simulink model "four"  (R2019b)
settings: Solver=VariableStepAuto  StartTime=0.0  StopTime=2  RelTol=1e-3
undefined symbols (not defined in the file): magnitude
libraries: dsparch4 x1
settings Model: Creator=Lenovo  LastModifiedBy=Lenovo

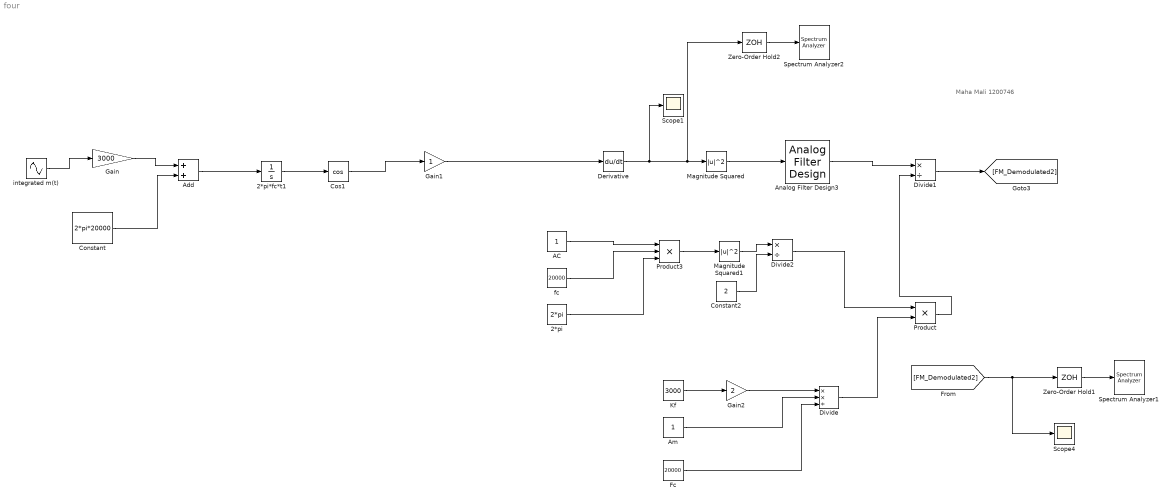
== system four ==
  note: Maha Mali 1200746
  2*pi : Constant  Value=2*pi
  2*pi*fc*t1 : Integrator
  AC : Constant
  Add : Sum
  Am : Constant
  Analog Filter Design3 : dsparch4/Analog Filter Design  method=Butterworth  filttype=Bandpass  N=8  Wlo=pi*2*400  Whi=pi*2*600  Rp=2  Rs=40
  Constant : Constant  Value=2*pi*20000
  Constant2 : Constant  Value=2
  Cos1 : Trigonometry  Operator=cos
  Derivative : Derivative
  Divide : Product  Inputs=**/
  Divide1 : Product  Inputs=*/
  Divide2 : Product  Inputs=*/
  Fc : Constant  Value=20000
  Gain : Gain  Gain=3000
  Gain1 : Gain
  Gain2 : Gain  Gain=2
  Kf : Constant  Value=3000
  Magnitude Squared : Math  Operator=magnitude^2  SignedPower=off  SaturateOnIntegerOverflow=on
  Magnitude Squared1 : Math  Operator=magnitude^2  SignedPower=off  SaturateOnIntegerOverflow=on
  Product : Product
  Product3 : Product  Inputs=3
  Scope1 : Scope
  Scope4 : Scope
  Spectrum Analyzer1 : SpectrumAnalyzer
  Spectrum Analyzer2 : SpectrumAnalyzer
  Zero-Order Hold1 : ZeroOrderHold  SampleTime=1/(10*5e2)
  Zero-Order Hold2 : ZeroOrderHold  SampleTime=1/(10*2e4)
  fc : Constant  Value=20000
  integrated m(t) : Sin  Frequency=500*pi*2  SampleTime=0
  wires:
  Product/1 -> Divide1/2
  Divide1/1 -> [FM_Demodulated2]
  fc/1 -> Product3/2
  Divide2/1 -> Product/1
  Fc/1 -> Divide/3
  Am/1 -> Divide/2
  [FM_Demodulated2] -> Zero-Order Hold1/1, Scope4/1
  AC/1 -> Product3/1
  Kf/1 -> Gain2/1
  2*pi/1 -> Product3/3
  Magnitude Squared1/1 -> Divide2/1
  Magnitude Squared/1 -> Analog Filter Design3/1
  Gain2/1 -> Divide/1
  Zero-Order Hold1/1 -> Spectrum Analyzer1/1
  Gain1/1 -> Derivative/1
  Analog Filter Design3/1 -> Divide1/1
  2*pi*fc*t1/1 -> Cos1/1
  Derivative/1 -> Scope1/1, Zero-Order Hold2/1, Magnitude Squared/1
  Add/1 -> 2*pi*fc*t1/1
  Gain/1 -> Add/1
  Product3/1 -> Magnitude Squared1/1
  Cos1/1 -> Gain1/1
  Constant2/1 -> Divide2/2
  Constant/1 -> Add/2
  integrated m(t)/1 -> Gain/1
  Divide/1 -> Product/2
  Zero-Order Hold2/1 -> Spectrum Analyzer2/1
